simulink model "Aircraft6dof_V2"  (R2025b)
settings: Solver=ode4  StartTime=startTime  StopTime=A8.stopTime  FixedStep=stepTime  RelTol=1e-3  EnableMultiTasking=on
undefined symbols (not defined in the file): a0_s2, a0_s3, a0_s4, a0_s5, A8, AR_s2, AR_s3, AR_s4, AR_s5, ARvecP1, Att_Trim, c_s2, c_s3, c_s4, c_s5, CD0_s2, CD0_s3, CD0_s4, CD0_s5, CDa_s2, CDa_s3, CDa_s4, CDa_s5, CL0_s2, CL0_s3, CL0_s4, CL0_s5, CM0_s2, CM0_s3, CM0_s4, CM0_s5, CMa_s2, CMa_s3, CMa_s4, CMa_s5, CQvecP1, CTvecP1, dCL_du, e_s2, e_s3, e_s4, e_s5, i_s2, i_s3, i_s4, i_s5, InitAtt, J, J_int, K_lqr_cmd, m, n_int, n_p1, n_s2, n_s3, n_s4, n_s5, R_p1, Rates_Trim, S_s2 ... (+15)
libraries: vrlib x9, simulink x5
(part 1 of 3)
settings Model: Creator=McArthur  LastModifiedBy=jacks
settings SolverCC: AlgebraicLoopSolver=TrustRegion
settings DataIOCC: LimitDataPoints=on  SaveFormat=StructureWithTime  ReturnWorkspaceOutputs=off
settings OptimizationCC: LifeSpan=inf
settings DebuggingCC: UnconnectedInputMsg=warning  UnconnectedOutputMsg=warning  UnconnectedLineMsg=warning  SFUnexpectedBacktrackingDiag=warning  SFNoUnconditionalDefaultTransitionDiag=warning  SFExecutionAtInitializationDiag=none  ArithmeticOperatorsInVariantConditions=warning
settings HardwareCC: ProdBitPerSizeT=32.0  ProdBitPerPtrDiffT=32.0  ProdWordSize=32.0  ProdHWDeviceType=Specified
settings ModelReferenceCC: EnableRefExpFcnMdlSchedulingChecks=on  PropagateSignalLabelsOutOfModel=off
settings SFSimCC: SimUseLocalCustomCode=off  CustomCodeUndefinedFunction=UseInterfaceOnly
settings RTWCC: RTWUseLocalCustomCode=off  GPUComputeCapability=3.5
settings CodeAppCC: StateflowObjectComments=on
settings GRTTargetCC: TargetLangStandard=C89/C90 (ANSI)
settings ConfigComp: CovMetricSettings=dw  CovSaveCumulativeToWorkspaceVar=on  CovSaveSingleToWorkspaceVar=on  CovExternalEMLEnable=off

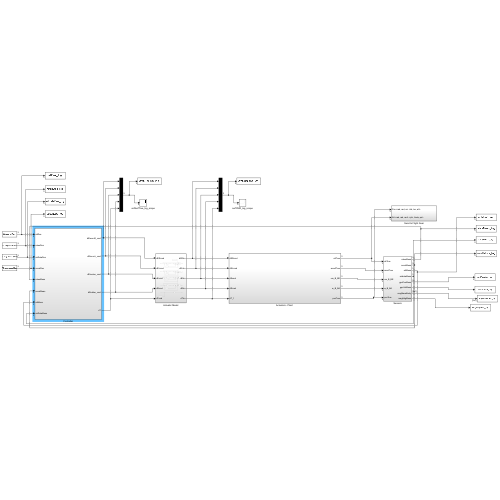
[thumbnail: Simulink's stored preview of the top-level diagram]
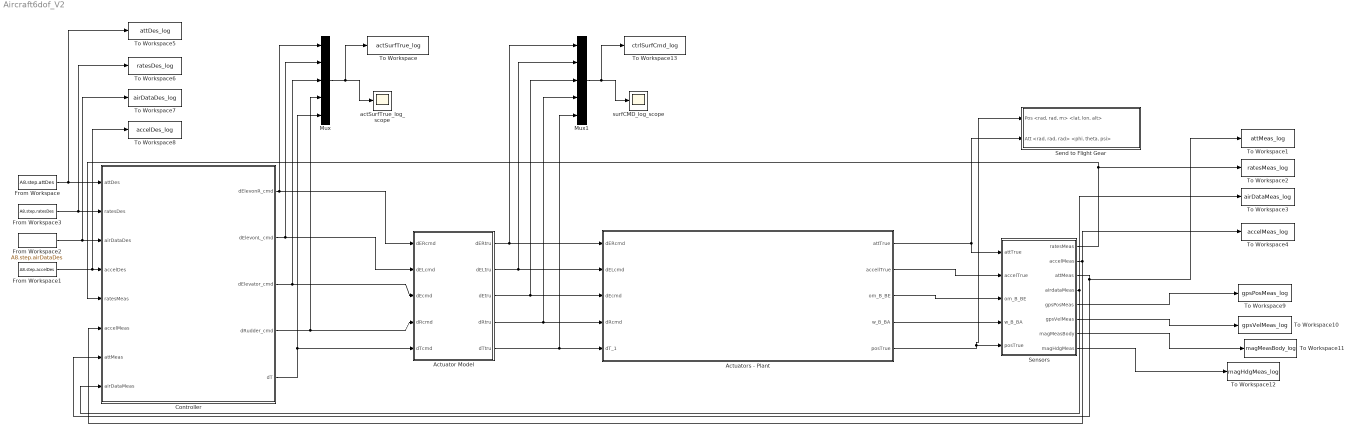
== system Aircraft6dof_V2 ==
  Actuator Model : Subsystem
  "Actuators - Plant " : Subsystem
  Controller : Subsystem
  From Workspace : FromWorkspace  VariableName=A8.step.attDes
  From Workspace1 : FromWorkspace  VariableName=A8.step.accelDes
  From Workspace2 : FromWorkspace  VariableName=A8.step.airDataDes
  From Workspace3 : FromWorkspace  VariableName=A8.step.ratesDes
  Mux : Mux  Inputs=5
  Mux1 : Mux  Inputs=5
  Send to Flight Gear : Subsystem
  Sensors : Subsystem
  To Workspace : ToWorkspace  VariableName=actSurfTrue_log  SaveFormat=Timeseries  SampleTime=-1
  To Workspace1 : ToWorkspace  VariableName=attMeas_log  SaveFormat=Timeseries  SampleTime=-1
  To Workspace10 : ToWorkspace  VariableName=gpsVelMeas_log  SaveFormat=Timeseries  SampleTime=-1
  To Workspace11 : ToWorkspace  VariableName=magMeasBody_log  SaveFormat=Timeseries  SampleTime=-1
  To Workspace12 : ToWorkspace  VariableName=magHdgMeas_log  SaveFormat=Timeseries  SampleTime=-1
  To Workspace13 : ToWorkspace  VariableName=ctrlSurfCmd_log  SaveFormat=Timeseries  SampleTime=-1
  To Workspace2 : ToWorkspace  VariableName=ratesMeas_log  SaveFormat=Timeseries  SampleTime=-1
  To Workspace3 : ToWorkspace  VariableName=airDataMeas_log  SaveFormat=Timeseries  SampleTime=-1
  To Workspace4 : ToWorkspace  VariableName=accelMeas_log  SaveFormat=Timeseries  SampleTime=-1
  To Workspace5 : ToWorkspace  VariableName=attDes_log  SaveFormat=Timeseries  SampleTime=-1
  To Workspace6 : ToWorkspace  VariableName=ratesDes_log  SaveFormat=Timeseries  SampleTime=-1
  To Workspace7 : ToWorkspace  VariableName=airDataDes_log  SaveFormat=Timeseries  SampleTime=-1
  To Workspace8 : ToWorkspace  VariableName=accelDes_log  SaveFormat=Timeseries  SampleTime=-1
  To Workspace9 : ToWorkspace  VariableName=gpsPosMeas_log  SaveFormat=Timeseries  SampleTime=-1
  actSurfTrue_log_scope : Scope
      settings: ActiveDisplayYMinimum=-0.54541539124822791  ActiveDisplayYMaximum=0.54541539124822791  DataLoggingVariableName=ScopeData24
  surfCMD_log_scope : Scope
      settings: ActiveDisplayYMinimum=-0.54541539124822791  ActiveDisplayYMaximum=0.54541539124822791  DataLoggingVariableName=ScopeData12
  wires:
  "Actuators - Plant "/5(posTrue) -> Send to Flight Gear/1("Pos <rad, rad, m> <lat, lon, alt>"), Sensors/5(posTrue)
  "Actuators - Plant "/4(w_B_BA) -> Sensors/4(w_B_BA)
  "Actuators - Plant "/3(om_B_BE) -> Sensors/3(om_B_BE)
  "Actuators - Plant "/2(accellTrue) -> Sensors/2(accelTrue)
  "Actuators - Plant "/1(attTrue) -> Send to Flight Gear/2("Att <rad, rad, rad> <phi, theta, psi>"), Sensors/1(attTrue)
  Controller/4(dRudder_cmd) -> Actuator Model/4(dRcmd), Mux/4
  Controller/3(dElevator_cmd) -> Actuator Model/3(dEcmd), Mux/3
  Controller/2(dElevonL_cmd) -> Actuator Model/2(dELcmd), Mux/2
  Controller/1(dElevonR_cmd) -> Actuator Model/1(dERcmd), Mux/1
  Sensors/1(ratesMeas) -> To Workspace2/1, Controller/5(ratesMeas)
  Sensors/3(attMeas) -> To Workspace1/1, Controller/7(attMeas)
  Sensors/2(accelMeas) -> Controller/6(accelMeas), To Workspace4/1
  Sensors/4(airdataMeas) -> Controller/8(airDataMeas), To Workspace3/1
  From Workspace1/1 -> To Workspace8/1, Controller/4(accelDes)
  From Workspace2/1 -> To Workspace7/1, Controller/3(airDataDes)
  From Workspace3/1 -> To Workspace6/1, Controller/2(ratesDes)
  Mux/1 -> actSurfTrue_log_scope/1, To Workspace/1
  Sensors/5(gpsPosMeas) -> To Workspace9/1
  Sensors/6(gpsVelMeas) -> To Workspace10/1
  Sensors/7(magMeasBody) -> To Workspace11/1
  Sensors/8(magHdgMeas) -> To Workspace12/1
  From Workspace/1 -> To Workspace5/1, Controller/1(attDes)
  Actuator Model/1(dERtru) -> Mux1/1, "Actuators - Plant "/1(dERcmd)
  Actuator Model/2(dELtru) -> Mux1/2, "Actuators - Plant "/2(dELcmd)
  Actuator Model/3(dEtru) -> Mux1/3, "Actuators - Plant "/3(dEcmd)
  Actuator Model/4(dRtru) -> Mux1/4, "Actuators - Plant "/4(dRcmd)
  Actuator Model/5(dTtru) -> Mux1/5, "Actuators - Plant "/5(dT_1)
  Controller/5(dT) -> Mux/5, Actuator Model/5(dTcmd)
  Mux1/1 -> surfCMD_log_scope/1, To Workspace13/1

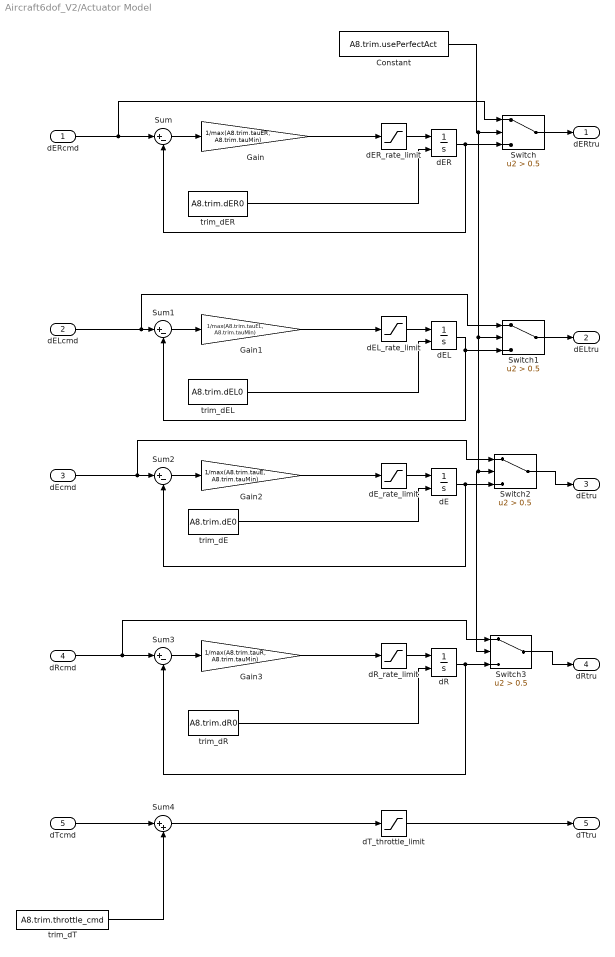
== system Aircraft6dof_V2/Actuator Model ==
  dERcmd : Inport
  dELcmd : Inport  Port=2
  dEcmd : Inport  Port=3
  dRcmd : Inport  Port=4
  dTcmd : Inport  Port=5
  Constant : Constant  Value=A8.trim.usePerfectAct
  Gain : Gain  Gain=1/max(A8.trim.tauER, A8.trim.tauMin)
  Gain1 : Gain  Gain=1/max(A8.trim.tauEL, A8.trim.tauMin)
  Gain2 : Gain  Gain=1/max(A8.trim.tauE, A8.trim.tauMin)
  Gain3 : Gain  Gain=1/max(A8.trim.tauR, A8.trim.tauMin)
  Sum{,1..3} (4 alike) : Sum  Inputs=|+-
  Sum4 : Sum  Inputs=|++
  Switch{,1..3} (4 alike) : Switch  Criteria=u2 > Threshold  Threshold=0.5  SaturateOnIntegerOverflow=off  InputSameDT=off
  dE : Integrator  InitialConditionSource=external  LimitOutput=on  UpperSaturationLimit=A8.trim.dE_max  LowerSaturationLimit=A8.trim.dE_min
  dEL : Integrator  InitialConditionSource=external  LimitOutput=on  UpperSaturationLimit=A8.trim.dEL_max  LowerSaturationLimit=A8.trim.dEL_min
  dEL_rate_limit : Saturate  UpperLimit=A8.trim.dELdot_max  LowerLimit=-A8.trim.dELdot_max
  dER : Integrator  InitialConditionSource=external  LimitOutput=on  UpperSaturationLimit=A8.trim.dER_max  LowerSaturationLimit=A8.trim.dER_min
  dER_rate_limit : Saturate  UpperLimit=A8.trim.dERdot_max  LowerLimit=-A8.trim.dERdot_max
  dE_rate_limit : Saturate  UpperLimit=A8.trim.dEdot_max  LowerLimit=-A8.trim.dEdot_max
  dR : Integrator  InitialConditionSource=external  LimitOutput=on  UpperSaturationLimit=A8.trim.dR_max  LowerSaturationLimit=A8.trim.dR_min
  dR_rate_limit : Saturate  UpperLimit=A8.trim.dRdot_max  LowerLimit=-A8.trim.dRdot_max
  dT_throttle_limit : Saturate  UpperLimit=A8.trim.dT1_max  LowerLimit=A8.trim.dT1_min
  trim_dE : Constant  Value=A8.trim.dE0
  trim_dEL : Constant  Value=A8.trim.dEL0
  trim_dER : Constant  Value=A8.trim.dER0
  trim_dR : Constant  Value=A8.trim.dR0
  trim_dT : Constant  Value=A8.trim.throttle_cmd
  dERtru : Outport  VectorParamsAs1DForOutWhenUnconnected=off
  dELtru : Outport  Port=2  VectorParamsAs1DForOutWhenUnconnected=off
  dEtru : Outport  Port=3  VectorParamsAs1DForOutWhenUnconnected=off
  dRtru : Outport  Port=4  VectorParamsAs1DForOutWhenUnconnected=off
  dTtru : Outport  Port=5
  wires:
  trim_dR/1 -> dR/2
  dER/1 -> Switch/3, Sum/2
  dE/1 -> Switch2/3, Sum2/2
  trim_dER/1 -> dER/2
  Gain1/1 -> dEL_rate_limit/1
  dERcmd/1 -> Switch/1, Sum/1
  Sum2/1 -> Gain2/1
  trim_dEL/1 -> dEL/2
  Gain/1 -> dER_rate_limit/1
  Gain3/1 -> dR_rate_limit/1
  trim_dE/1 -> dE/2
  dRcmd/1 -> Switch3/1, Sum3/1
  Gain2/1 -> dE_rate_limit/1
  Sum1/1 -> Gain1/1
  Sum/1 -> Gain/1
  Sum3/1 -> Gain3/1
  dELcmd/1 -> Switch1/1, Sum1/1
  dEcmd/1 -> Switch2/1, Sum2/1
  dEL/1 -> Switch1/3, Sum1/2
  dR/1 -> Switch3/3, Sum3/2
  dT_throttle_limit/1 -> dTtru/1
  dTcmd/1 -> Sum4/1
  trim_dT/1 -> Sum4/2
  dER_rate_limit/1 -> dER/1
  dEL_rate_limit/1 -> dEL/1
  dE_rate_limit/1 -> dE/1
  dR_rate_limit/1 -> dR/1
  Sum4/1 -> dT_throttle_limit/1
  Switch/1 -> dERtru/1
  Constant/1 -> Switch3/2, Switch2/2, Switch1/2, Switch/2
  Switch1/1 -> dELtru/1
  Switch2/1 -> dEtru/1
  Switch3/1 -> dRtru/1

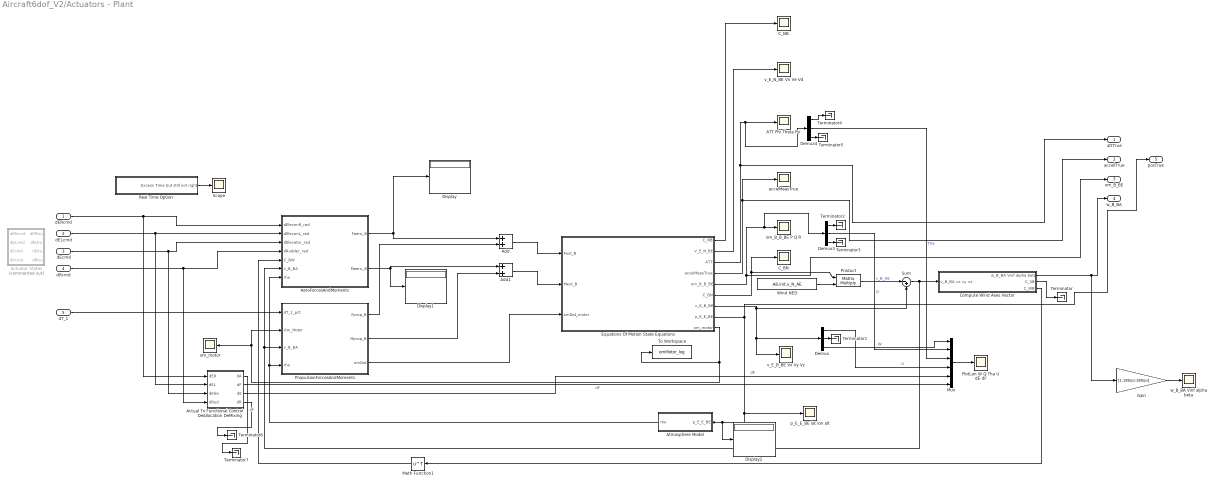
== system Aircraft6dof_V2/Actuators - Plant  ==
  dERcmd : Inport
  dELcmd : Inport  Port=2
  dEcmd : Inport  Port=3
  dRcmd : Inport  Port=4
  dT_1 : Inport  Port=5
  ATT Phi Theta Psi : Scope
      settings: TimeSpan=100  ActiveDisplayYMinimum=-0.03536052016506628  ActiveDisplayYMaximum=0.060071284999749723  DataLoggingVariableName=ScopeData6
  Actual To Functional Control DeAllocation DeMixing : Subsystem
  Actuator States : Subsystem  Commented=on
  Add : Sum
  Add1 : Sum
  AeroForcesAndMoments : Subsystem
  Atmosphere Model : Subsystem
  C_BN : Scope
      settings: ActiveDisplayYMinimum=-1.25  ActiveDisplayYMaximum=1.25  DataLoggingVariableName=ScopeData7
  C_NB : Scope
      settings: DataLoggingVariableName=ScopeData8  DataLoggingSaveFormat=Array
  Compute Wind Axes Vector : Subsystem
  Demux : Demux  Outputs=3
  Demux3 : Demux  Outputs=3
  Demux4 : Demux  Outputs=3
  Display : Display
  Display1 : Display
  Display2 : Display
  Equations Of Motion State Equations : Subsystem
  Gain : Gain  Gain=[1;180/pi;180/pi]
  Math Function1 : Math  Operator=transpose  SignedPower=on
  Mux : Mux  Inputs=6
  PlotLon W Q Tha U dE dF : Scope
      settings: TimeSpan=100  ActiveDisplayYMinimum=-109.39087703202826  ActiveDisplayYMaximum=114.84829731514765  DataLoggingVariableName=ScopeData11
  Product : Product  Multiplication=Matrix(*)
  PropulsionForcesAndMoments : Subsystem
  Real Time Option : Subsystem
  Scope : Scope
      settings: ActiveDisplayYMinimum=-0.02501  ActiveDisplayYMaximum=0.00268
  Sum : Sum  Inputs=|-+
  Terminator{,1..7} (8 alike) : Terminator
  To Workspace : ToWorkspace  VariableName=omMotor_log  SaveFormat=Timeseries  SampleTime=-1
  Wind NED : Constant  Value=A8.init.v_N_AE
  accelMeasTrue : Scope
      settings: TimeSpan=20  ActiveDisplayYMinimum=-12  ActiveDisplayYMaximum=3  DataLoggingVariableName=ScopeData5  DataLoggingSaveFormat=Array
  om_B_B_BE P Q R : Scope
      settings: TimeSpan=20  ActiveDisplayYMinimum=-0.175  ActiveDisplayYMaximum=0.125  DataLoggingVariableName=ScopeData4
  om_motor : Scope
      settings: TimeSpan=20  ActiveDisplayYMinimum=-1  ActiveDisplayYMaximum=1  DataLoggingVariableName=ScopeData2
  p_E_E_BE lat lon alt : Scope
      settings: ActiveDisplayYMinimum=-2197.24995  ActiveDisplayYMaximum=255.24999
  v_E_B_BE Vx Vy Vz : Scope
      settings: TimeSpan=20  ActiveDisplayYMinimum=-95.74229  ActiveDisplayYMaximum=24.82944  DataLoggingVariableName=ScopeData3
  v_E_N_BE Vn Ve Vd : Scope
      settings: TimeSpan=20  ActiveDisplayYMinimum=-27.392800404423681  ActiveDisplayYMaximum=39.4717463834183  DataLoggingVariableName=ScopeData9  DataLoggingSaveFormat=Array
  w_B_BA Vinf alpha beta : Scope
      settings: TimeSpan=20  ActiveDisplayYMinimum=-1  ActiveDisplayYMaximum=1  DataLoggingVariableName=ScopeData10
  attTrue : Outport
  accellTrue : Outport  Port=2
  om_B_BE : Outport  Port=3
  w_B_BA : Outport  Port=4
  posTrue : Outport  Port=5
  wires:
  Real Time Option/1(Excess Time but still not right) -> Scope/1
  AeroForcesAndMoments/2(Maero_B) -> Add1/1, Display1/1
  PropulsionForcesAndMoments/3(omDot) -> Equations Of Motion State Equations/3(omDot_motor)
  AeroForcesAndMoments/1(Faero_B) -> Add/1, Display/1
  Equations Of Motion State Equations/8(p_E_E_BE) -> Display2/1, Atmosphere Model/1(p_E_E_BE), p_E_E_BE lat lon alt/1, posTrue/1
  Equations Of Motion State Equations/2(V_E_N_BE) -> v_E_N_BE Vn Ve Vd/1
  Equations Of Motion State Equations/1(C_NB) -> C_NB/1
  Sum/1 -> PropulsionForcesAndMoments/3(v_B_BA), AeroForcesAndMoments/6(v_B_BA), Compute Wind Axes Vector/1(v_B_BA vx vy vz)
  Compute Wind Axes Vector/3(C_WB) -> Math Function1/1
  Math Function1/1 -> AeroForcesAndMoments/5(C_BW)
  Equations Of Motion State Equations/5(om_B_B_BE) -> Demux3/1, om_B_B_BE P Q R/1, om_B_BE/1
  Equations Of Motion State Equations/6(C_BN) -> C_BN/1, Product/1
  Product/1 -> Sum/1  "v_B_AE"
  Gain/1 -> w_B_BA Vinf alpha beta/1
  Atmosphere Model/1(rho) -> PropulsionForcesAndMoments/4(rho), AeroForcesAndMoments/7(rho)
  Compute Wind Axes Vector/1(w_B_BA Vinf alpha beta) -> Gain/1, w_B_BA/1
  Compute Wind Axes Vector/2(C_SB) -> Terminator/1
  Equations Of Motion State Equations/7(v_E_B_BE) -> Sum/2, v_E_B_BE Vx Vy Vz/1, Demux/1
  Equations Of Motion State Equations/4(accelMeasTrue) -> accellTrue/1, accelMeasTrue/1
  Wind NED/1 -> Product/2
  Mux/1 -> PlotLon W Q Tha U dE dF/1
  Demux/3 -> Mux/1  "W"
  Demux/1 -> Mux/4  "U"
  Demux/2 -> Terminator1/1
  Demux3/2 -> Mux/2  "Q"
  Demux3/1 -> Terminator2/1
  Demux3/3 -> Terminator3/1
  Equations Of Motion State Equations/3(ATT) -> Demux4/1, ATT Phi Theta Psi/1, attTrue/1
  Demux4/2 -> Mux/3  "Tha"
  Demux4/1 -> Terminator4/1
  Demux4/3 -> Terminator5/1
  Actual To Functional Control DeAllocation DeMixing/3(dE) -> Mux/5  "dE"
  Actual To Functional Control DeAllocation DeMixing/2(dF) -> Mux/6  "dF"
  Add/1 -> Equations Of Motion State Equations/1(Fext_B)
  Add1/1 -> Equations Of Motion State Equations/2(Mext_B)
  dT_1/1 -> PropulsionForcesAndMoments/1(dT_1_pct)
  PropulsionForcesAndMoments/1(Fprop_B) -> Add/2
  PropulsionForcesAndMoments/2(Mprop_B) -> Add1/2
  Equations Of Motion State Equations/9(om_motor) -> To Workspace/1, PropulsionForcesAndMoments/2(Om_Motor), om_motor/1
  Actual To Functional Control DeAllocation DeMixing/4(dR) -> Terminator6/1
  Actual To Functional Control DeAllocation DeMixing/1(dA) -> Terminator7/1  "dF"
  dERcmd/1 -> Actual To Functional Control DeAllocation DeMixing/1(dER), AeroForcesAndMoments/1(dElevonR_rad)
  dELcmd/1 -> Actual To Functional Control DeAllocation DeMixing/2(dEL), AeroForcesAndMoments/2(dElevonL_rad)
  dEcmd/1 -> Actual To Functional Control DeAllocation DeMixing/3(dElev), AeroForcesAndMoments/3(dElevator_rad)
  dRcmd/1 -> Actual To Functional Control DeAllocation DeMixing/4(dRud), AeroForcesAndMoments/4(dRudder_rad)

== system Aircraft6dof_V2/Controller ==
  attDes : Inport
  ratesDes : Inport  Port=2
  airDataDes : Inport  Port=3
  accelDes : Inport  Port=4
  ratesMeas : Inport  Port=5
  accelMeas : Inport  Port=6
  attMeas : Inport  Port=7
  airDataMeas : Inport  Port=8
  Constant1 : Constant  Value=A8.gains.on
  ControlMixer_A8 : Subsystem
  Demux : Demux  Outputs=5
  LQR Controller : Subsystem
  Multiport Switch : MultiPortSwitch  SaturateOnIntegerOverflow=off  InputSameDT=off
  Mux : Mux  Inputs=5
  Mux1 : Mux  Inputs=5
  Mux2 : Mux  Inputs=5
  "No Feedback Open Loop Commands Steps, Ramps, Sweeps, etc" : Subsystem
  PID Controller : Subsystem
  To Workspace : ToWorkspace  VariableName=ctrlFunc_log  SaveFormat=Timeseries  SampleTime=-1
  dElevonR_cmd : Outport  VectorParamsAs1DForOutWhenUnconnected=off
  dElevonL_cmd : Outport  Port=2  VectorParamsAs1DForOutWhenUnconnected=off
  dElevator_cmd : Outport  Port=3  VectorParamsAs1DForOutWhenUnconnected=off
  dRudder_cmd : Outport  Port=4  VectorParamsAs1DForOutWhenUnconnected=off
  dT : Outport  Port=5  VectorParamsAs1DForOutWhenUnconnected=off
  wires:
  accelMeas/1 -> "No Feedback Open Loop Commands Steps, Ramps, Sweeps, etc"/8(accelMeas), PID Controller/8(accelMeas)
  attDes/1 -> LQR Controller/4(attDes), PID Controller/1(attDes), "No Feedback Open Loop Commands Steps, Ramps, Sweeps, etc"/1(attDes)
  ratesMeas/1 -> LQR Controller/2(ratesMeas), "No Feedback Open Loop Commands Steps, Ramps, Sweeps, etc"/6(ratesMeas), PID Controller/6(ratesMeas)
  ratesDes/1 -> LQR Controller/5(ratesDes), "No Feedback Open Loop Commands Steps, Ramps, Sweeps, etc"/2(ratesDes), PID Controller/2(ratesDes)
  attMeas/1 -> LQR Controller/1(attMeas), "No Feedback Open Loop Commands Steps, Ramps, Sweeps, etc"/5(attMeas), PID Controller/5(attMeas)
  Demux/1 -> ControlMixer_A8/1(dA)
  airDataDes/1 -> LQR Controller/6(airDataDes), "No Feedback Open Loop Commands Steps, Ramps, Sweeps, etc"/3(airDataDes), PID Controller/3(airDataDes)
  accelDes/1 -> "No Feedback Open Loop Commands Steps, Ramps, Sweeps, etc"/4(accelDes), PID Controller/4(accelDes)
  airDataMeas/1 -> LQR Controller/3(airDataMeas), "No Feedback Open Loop Commands Steps, Ramps, Sweeps, etc"/7(airDataMeas), PID Controller/7(airDataMeas)
  ControlMixer_A8/2(dELcmd) -> dElevonL_cmd/1
  "No Feedback Open Loop Commands Steps, Ramps, Sweeps, etc"/1(dAil) -> Mux/1
  "No Feedback Open Loop Commands Steps, Ramps, Sweeps, etc"/4(dRud) -> Mux/4
  "No Feedback Open Loop Commands Steps, Ramps, Sweeps, etc"/3(dElev) -> Mux/3
  "No Feedback Open Loop Commands Steps, Ramps, Sweeps, etc"/2(dFlap) -> Mux/2
  "No Feedback Open Loop Commands Steps, Ramps, Sweeps, etc"/5(dT) -> Mux/5
  PID Controller/4(dRud) -> Mux1/4
  PID Controller/3(dElev) -> Mux1/3
  PID Controller/2(dFlap) -> Mux1/2
  PID Controller/1(dAil) -> Mux1/1
  PID Controller/5(dT) -> Mux1/5
  Mux/1 -> Multiport Switch/2
  Demux/5 -> ControlMixer_A8/5(dT)
  Demux/4 -> ControlMixer_A8/4(dR)
  Demux/3 -> ControlMixer_A8/3(dE)
  Demux/2 -> ControlMixer_A8/2(dF)
  ControlMixer_A8/1(dERcmd) -> dElevonR_cmd/1
  ControlMixer_A8/3(dElevcmd) -> dElevator_cmd/1
  ControlMixer_A8/4(dRudcmd) -> dRudder_cmd/1
  ControlMixer_A8/5(dTcmd) -> dT/1
  Constant1/1 -> Multiport Switch/1
  Mux1/1 -> Multiport Switch/3
  LQR Controller/4(dRud) -> Mux2/4
  LQR Controller/5(dT) -> Mux2/5
  LQR Controller/3(dElev) -> Mux2/3
  LQR Controller/2(dFlap) -> Mux2/2
  LQR Controller/1(dAil) -> Mux2/1
  Mux2/1 -> Multiport Switch/4
  Multiport Switch/1 -> To Workspace/1, Demux/1

== system Aircraft6dof_V2/Send to Flight Gear ==
  "Pos <rad, rad, m> <lat, lon, alt>" : Inport
  "Att <rad, rad, rad> <phi, theta, psi>" : Inport  Port=2
  S-Function : S-Function  FunctionName=sfun_FlightGearSender  Parameters=stepTime, '127.0.0.1', 5502  SFunctionDeploymentMode=off  EnableBusSupport=off
  wires:
  "Pos <rad, rad, m> <lat, lon, alt>"/1 -> S-Function/1
  "Att <rad, rad, rad> <phi, theta, psi>"/1 -> S-Function/2

== system Aircraft6dof_V2/Sensors ==
  attTrue : Inport
  accelTrue : Inport  Port=2
  om_B_BE : Inport  Port=3
  w_B_BA : Inport  Port=4
  posTrue : Inport  Port=5
  AccelSensor : Subsystem
  AirDataSensor : Subsystem
  AttitudeSensor : Subsystem
  GPSSensor : Subsystem
  GyroSensor : Subsystem
  MagSensor : Subsystem
  Selector : Selector  InputPortWidth=3  IndexOptions=Index vector (dialog)  Indices=[1]  OutputSizes=1
  ratesMeas : Outport  VectorParamsAs1DForOutWhenUnconnected=off
  accelMeas : Outport  Port=2  VectorParamsAs1DForOutWhenUnconnected=off
  attMeas : Outport  Port=3  VectorParamsAs1DForOutWhenUnconnected=off
  airdataMeas : Outport  Port=4
  gpsPosMeas : Outport  Port=5
  gpsVelMeas : Outport  Port=6
  magMeasBody : Outport  Port=7
  magHdgMeas : Outport  Port=8
  wires:
  AccelSensor/1(accelMeas) -> accelMeas/1
  accelTrue/1 -> AccelSensor/1(accelTrue)
  attTrue/1 -> AttitudeSensor/1(attTrue), MagSensor/1(attTrue)
  GyroSensor/1(ratesMeas) -> ratesMeas/1
  Selector/1 -> GPSSensor/2(velTrue)
  w_B_BA/1 -> AirDataSensor/1(w_B_BA), Selector/1
  om_B_BE/1 -> GyroSensor/1(ratesTrue)
  AttitudeSensor/1(attMeas) -> attMeas/1
  MagSensor/1(magMeasBody) -> magMeasBody/1
  MagSensor/2(magHdgMeas) -> magHdgMeas/1
  posTrue/1 -> GPSSensor/1(posTrue)
  AirDataSensor/1(airdataMeas) -> airdataMeas/1
  GPSSensor/2(gpsVelMeas) -> gpsVelMeas/1
  GPSSensor/1(gpsPosMeas) -> gpsPosMeas/1

== system Aircraft6dof_V2/Actuators - Plant /Actual To Functional Control DeAllocation DeMixing ==
  dER : Inport
  dEL : Inport  Port=2
  dElev : Inport  Port=3
  dRud : Inport  Port=4
  Constant1 : Constant  Value=A8.trim.DeMixMatrix
  Demux : Demux
  Mux : Mux
  Product1 : Product  Multiplication=Matrix(*)
  dA : Outport  VectorParamsAs1DForOutWhenUnconnected=off
  dF : Outport  Port=2  VectorParamsAs1DForOutWhenUnconnected=off
  dE : Outport  Port=3  VectorParamsAs1DForOutWhenUnconnected=off
  dR : Outport  Port=4  VectorParamsAs1DForOutWhenUnconnected=off
  wires:
  dER/1 -> Mux/1
  dEL/1 -> Mux/2
  dElev/1 -> Mux/3
  dRud/1 -> Mux/4
  Demux/2 -> dF/1
  Constant1/1 -> Product1/1
  Mux/1 -> Product1/2
  Demux/1 -> dA/1
  Demux/4 -> dR/1
  Demux/3 -> dE/1
  Product1/1 -> Demux/1

== system Aircraft6dof_V2/Actuators - Plant /Actuator States ==
  dERcmd : Inport
  dELcmd : Inport  Port=2
  dEcmd : Inport  Port=3
  dRcmd : Inport  Port=4
  Gain : Gain  Gain=1/A8.trim.tauER
  Gain1 : Gain  Gain=1/A8.trim.tauEL
  Gain2 : Gain  Gain=1/A8.trim.tauE
  Gain3 : Gain  Gain=1/A8.trim.tauR
  Sum{,1..3} (4 alike) : Sum  Inputs=|+-
  dE : Integrator  InitialConditionSource=external
  dEL : Integrator  InitialConditionSource=external
  dER : Integrator  InitialConditionSource=external
  dR : Integrator  InitialConditionSource=external
  trim_dE : Constant  Value=A8.trim.dE0
  trim_dEL : Constant  Value=A8.trim.dEL0
  trim_dER : Constant  Value=A8.trim.dER0
  trim_dR : Constant  Value=A8.trim.dR0
  dERtru : Outport  VectorParamsAs1DForOutWhenUnconnected=off
  dELtru : Outport  Port=2  VectorParamsAs1DForOutWhenUnconnected=off
  dEtru : Outport  Port=3  VectorParamsAs1DForOutWhenUnconnected=off
  dRtru : Outport  Port=4  VectorParamsAs1DForOutWhenUnconnected=off
  wires:
  dER/1 -> Sum/2, dERtru/1
  dERcmd/1 -> Sum/1
  Gain/1 -> dER/1
  Sum/1 -> Gain/1
  trim_dER/1 -> dER/2
  dEL/1 -> Sum1/2, dELtru/1
  dELcmd/1 -> Sum1/1
  Gain1/1 -> dEL/1
  Sum1/1 -> Gain1/1
  trim_dEL/1 -> dEL/2
  dE/1 -> Sum2/2, dEtru/1
  dEcmd/1 -> Sum2/1
  Gain2/1 -> dE/1
  Sum2/1 -> Gain2/1
  trim_dE/1 -> dE/2
  dR/1 -> Sum3/2, dRtru/1
  dRcmd/1 -> Sum3/1
  Gain3/1 -> dR/1
  Sum3/1 -> Gain3/1
  trim_dR/1 -> dR/2

== system Aircraft6dof_V2/Actuators - Plant /AeroForcesAndMoments ==
  dElevonR_rad : Inport
  dElevonL_rad : Inport  Port=2
  dElevator_rad : Inport  Port=3
  dRudder_rad : Inport  Port=4
  C_BW : Inport  Port=5
  v_B_BA : Inport  Port=6
  rho : Inport  Port=7
  Add : Sum  Inputs=++++
  Add1 : Sum  Inputs=++++
  Display1 : Display
  Display3 : Display
  Surface2 : Subsystem
  Surface3 : Subsystem
  Surface4 : Subsystem
  Surface5 : Subsystem
  Faero_B : Outport  VectorParamsAs1DForOutWhenUnconnected=off
  Maero_B : Outport  Port=2  VectorParamsAs1DForOutWhenUnconnected=off
  wires:
  C_BW/1 -> Surface2/1(C_BW), Surface3/1(C_BW), Surface5/1(C_BW), Surface4/1(C_BW)
  v_B_BA/1 -> Surface3/2(v_B_BA), Surface2/2(v_B_BA), Surface5/2(v_B_BA), Surface4/2(v_B_BA)
  rho/1 -> Surface3/3(rho), Surface2/3(rho), Surface5/3(rho), Surface4/3(rho)
  Surface4/1(Fs4_B) -> Add/1
  Surface5/1(Fs5_B) -> Add/2
  Surface4/2(Ms4_B) -> Add1/1
  Surface5/2(Ms5_B) -> Add1/2
  Surface2/1(Fs2_B) -> Add/3
  Surface2/2(Ms2_B) -> Add1/3
  Add1/1 -> Display1/1, Maero_B/1
  Add/1 -> Display3/1, Faero_B/1
  Surface3/1(Fs2_B) -> Add/4
  Surface3/2(Ms2_B) -> Add1/4
  dElevonR_rad/1 -> Surface4/4(u_s#_rad)
  dElevonL_rad/1 -> Surface5/4(u_s#_rad)
  dElevator_rad/1 -> Surface2/4(u_s#_rad)
  dRudder_rad/1 -> Surface3/4(u_s#_rad)

== system Aircraft6dof_V2/Actuators - Plant /Atmosphere Model ==
  p_E_E_BE : Inport
  Compare To Constant : simulink/Logic and Bit Operations/Compare To Constant  relop=<=  const=11000  OutDataTypeStr=boolean
  Demux : Demux  Outputs=3
  Enhance Me Please! : Constant  Value=0
  Standard Atmosphere - Troposphere : MATLAB Function  TreatAsAtomicUnit=on
  Switch : Switch  Criteria=u2 ~= 0  Threshold=11000  SaturateOnIntegerOverflow=off  InputSameDT=off
  Terminator : Terminator
  Terminator1 : Terminator
  rho : Outport  VectorParamsAs1DForOutWhenUnconnected=off
  wires:
  p_E_E_BE/1 -> Demux/1
  Demux/1 -> Terminator/1
  Demux/2 -> Terminator1/1
  Demux/3 -> Standard Atmosphere - Troposphere/1(h), Compare To Constant/1
  Compare To Constant/1 -> Switch/2
  Standard Atmosphere - Troposphere/1(rho) -> Switch/1
  Switch/1 -> rho/1
  Enhance Me Please!/1 -> Switch/3

== system Aircraft6dof_V2/Actuators - Plant /Compute Wind Axes Vector ==
  v_B_BA vx vy vz : Inport
  Compute Wind DCMs : MATLAB Function  TreatAsAtomicUnit=on
  Constant : Constant  Value=[0;0;0]
  Constant1 : Constant  Value=0.001
  Demux : Demux  Outputs=3
  Display : Display
  Divide : Product  Inputs=*/
  Dot Product : DotProduct  OutDataTypeStr=Inherit: Inherit via internal rule
  MinMax : MinMax  Function=max  Inputs=2
  Mux : Mux  Inputs=3
  Saturation : Saturate  UpperLimit=1  LowerLimit=-1
  Sqrt : Sqrt
  Switch : Switch  Criteria=u2 > Threshold  SaturateOnIntegerOverflow=off  InputSameDT=off
  Trigonometric Function : Trigonometry  Operator=atan2
  Trigonometric Function1 : Trigonometry  Operator=asin
  w_B_BA Vinf alpha beta : Outport  VectorParamsAs1DForOutWhenUnconnected=off
  C_SB : Outport  Port=2  VectorParamsAs1DForOutWhenUnconnected=off
  C_WB : Outport  Port=3  VectorParamsAs1DForOutWhenUnconnected=off
  wires:
  Dot Product/1 -> Sqrt/1
  Mux/1 -> Switch/1
  Constant/1 -> Switch/3
  Trigonometric Function/1 -> Display/1, Compute Wind DCMs/2(alpha), Mux/2
  Switch/1 -> w_B_BA Vinf alpha beta/1
  Demux/3 -> Trigonometric Function/1
  v_B_BA vx vy vz/1 -> Demux/1, Dot Product/2, Dot Product/1
  Demux/1 -> Trigonometric Function/2
  Constant1/1 -> MinMax/1
  MinMax/1 -> Divide/2
  Demux/2 -> Divide/1
  Divide/1 -> Saturation/1
  Saturation/1 -> Trigonometric Function1/1
  Trigonometric Function1/1 -> Compute Wind DCMs/3(beta), Mux/3
  Sqrt/1 -> Compute Wind DCMs/1(Vinf), Mux/1, Switch/2, MinMax/2
  Compute Wind DCMs/2(C_WB) -> C_WB/1
  Compute Wind DCMs/1(C_SB) -> C_SB/1

== system Aircraft6dof_V2/Actuators - Plant /Equations Of Motion State Equations ==
  Fext_B : Inport
  Mext_B : Inport  Port=2
  omDot_motor : Inport  Port=3
  Earth Model : Subsystem
  MATLAB Function : MATLAB Function  Commented=on  TreatAsAtomicUnit=on
  Math Function : Math  Operator=transpose  SignedPower=on
  Product1 : Product  Multiplication=Matrix(*)
  Product2 : Product  Multiplication=Matrix(*)
  QUAT2ATT : Subsystem
  QUAT2DCM : Subsystem
  Rot Dyn (Moments) : Subsystem
  Rot Kin (Orientation) Euler : Subsystem  Commented=on
  Rot Kin (Orientation) Quaternion : Subsystem
  Trans Dyn (Forces) : Subsystem
  Trans Kin (Spherical) : Subsystem
  C_NB : Outport  VectorParamsAs1DForOutWhenUnconnected=off
  V_E_N_BE : Outport  Port=2  VectorParamsAs1DForOutWhenUnconnected=off
  ATT : Outport  Port=3  VectorParamsAs1DForOutWhenUnconnected=off
  accelMeasTrue : Outport  Port=4  VectorParamsAs1DForOutWhenUnconnected=off
  om_B_B_BE : Outport  Port=5  VectorParamsAs1DForOutWhenUnconnected=off
  C_BN : Outport  Port=6  VectorParamsAs1DForOutWhenUnconnected=off
  v_E_B_BE : Outport  Port=7  VectorParamsAs1DForOutWhenUnconnected=off
  p_E_E_BE : Outport  Port=8  VectorParamsAs1DForOutWhenUnconnected=off
  om_motor : Outport  Port=9  VectorParamsAs1DForOutWhenUnconnected=off
  wires:
  omDot_motor/1 -> Rot Dyn (Moments)/2(omDot_motor)
  Rot Dyn (Moments)/1(om_B_B_BE) -> Trans Dyn (Forces)/3(om_B_B_BE), Rot Kin (Orientation) Quaternion/1(om_B_B_BN), Rot Kin (Orientation) Euler/1(om_B_B_BN), om_B_B_BE/1
  Trans Dyn (Forces)/1(xDot_E_B_BE) -> Trans Kin (Spherical)/1(v_E_B_BE), v_E_B_BE/1, Product1/2
  Rot Kin (Orientation) Quaternion/1(q_BN) -> QUAT2DCM/1(Quat), QUAT2ATT/1(q)
  QUAT2DCM/1(DCM) -> C_BN/1, Math Function/1, Product2/1  "C_BN"
  Mext_B/1 -> Rot Dyn (Moments)/1(Mext_B)
  Fext_B/1 -> Trans Dyn (Forces)/1(Fext_B)
  QUAT2ATT/1(ATT) -> MATLAB Function/1(ATT), ATT/1
  Trans Kin (Spherical)/1(p_E_E_BE) -> Earth Model/1(p_E_E_BE), p_E_E_BE/1
  Math Function/1 -> C_NB/1, Trans Kin (Spherical)/2(C_NB), Product1/1  "C_NB"
  Product1/1 -> V_E_N_BE/1
  Earth Model/2(g_N) -> Product2/2
  Product2/1 -> Trans Dyn (Forces)/2(g_B)
  Rot Dyn (Moments)/2(om_motor) -> om_motor/1
  Trans Dyn (Forces)/2(accelMeasCG) -> accelMeasTrue/1
  Earth Model/1(Rearth) -> Trans Kin (Spherical)/3(Rearth)

== system Aircraft6dof_V2/Actuators - Plant /PropulsionForcesAndMoments ==
  dT_1_pct : Inport
  Om_Motor : Inport  Port=2
  v_B_BA : Inport  Port=3
  rho : Inport  Port=4
  Add : Sum  Inputs=++++
  Add1 : Sum  Inputs=++++
  Constant : Constant  Value=0
  Display1 : Display
  Display3 : Display
  PropulsionSystem1 : Subsystem
  Fprop_B : Outport  VectorParamsAs1DForOutWhenUnconnected=off
  Mprop_B : Outport  Port=2  VectorParamsAs1DForOutWhenUnconnected=off
  omDot : Outport  Port=3  VectorParamsAs1DForOutWhenUnconnected=off
  wires:
  dT_1_pct/1 -> PropulsionSystem1/4(u_p#_pct)
  Add/1 -> Fprop_B/1, Display3/1
  Add1/1 -> Mprop_B/1, Display1/1
  Constant/1 -> Add1/4, Add1/3, Add1/2, Add/4, Add/3, Add/2
  PropulsionSystem1/1(Fs4_B) -> Add/1
  rho/1 -> PropulsionSystem1/3(rho)
  v_B_BA/1 -> PropulsionSystem1/2(v_B_BA)
  Om_Motor/1 -> PropulsionSystem1/1(Om_p1)
  PropulsionSystem1/2(Ms4_B) -> Add1/1
  PropulsionSystem1/3(omDot) -> omDot/1

== system Aircraft6dof_V2/Actuators - Plant /Real Time Option ==
  Timer for Real-Time : S-Function  FunctionName=sfun_RealTimeOptional  Parameters=RatioToRealTime  SFunctionDeploymentMode=off  EnableBusSupport=off
  Excess Time but still not right : Outport  VectorParamsAs1DForOutWhenUnconnected=off
  wires:
  Timer for Real-Time/1 -> Excess Time but still not right/1

== system Aircraft6dof_V2/Controller/ControlMixer_A8 ==
  dA : Inport
  dF : Inport  Port=2
  dE : Inport  Port=3
  dR : Inport  Port=4
  dT : Inport  Port=5
  Constant1 : Constant  Value=A8.trim.MixMatrix
  Demux : Demux
  Mux1 : Mux
  Product1 : Product  Multiplication=Matrix(*)
  Sum{,1,3..4} (4 alike) : Sum  Inputs=|++
  trim_dE : Constant  Value=A8.trim.dE0
  trim_dEL : Constant  Value=A8.trim.dEL0
  trim_dER : Constant  Value=A8.trim.dER0
  trim_dR : Constant  Value=A8.trim.dR0
  dERcmd : Outport  VectorParamsAs1DForOutWhenUnconnected=off
  dELcmd : Outport  Port=2  VectorParamsAs1DForOutWhenUnconnected=off
  dElevcmd : Outport  Port=3  VectorParamsAs1DForOutWhenUnconnected=off
  dRudcmd : Outport  Port=4  VectorParamsAs1DForOutWhenUnconnected=off
  dTcmd : Outport  Port=5
  wires:
  trim_dE/1 -> Sum3/2
  dA/1 -> Mux1/1
  Constant1/1 -> Product1/1
  dF/1 -> Mux1/2
  dE/1 -> Mux1/3
  Mux1/1 -> Product1/2
  dR/1 -> Mux1/4
  dT/1 -> dTcmd/1
  trim_dEL/1 -> Sum1/2
  Product1/1 -> Demux/1
  trim_dER/1 -> Sum/2
  Demux/1 -> Sum/1
  Demux/2 -> Sum1/1
  Demux/3 -> Sum3/1
  Demux/4 -> Sum4/1
  trim_dR/1 -> Sum4/2
  Sum/1 -> dERcmd/1
  Sum1/1 -> dELcmd/1
  Sum3/1 -> dElevcmd/1
  Sum4/1 -> dRudcmd/1

== system Aircraft6dof_V2/Controller/LQR Controller ==
  attMeas : Inport
  ratesMeas : Inport  Port=2
  airDataMeas : Inport  Port=3
  attDes : Inport  Port=4
  ratesDes : Inport  Port=5
  airDataDes : Inport  Port=6
  1 if doing test : Constant  Value=A8.step.useCMDs
  Constant2 : Constant  Value=0
  Demux : Demux
  Demux{1..2,4..5} (4 alike) : Demux  Outputs=3
  LQR_Gain : Gain  Gain=-K_lqr_cmd  Multiplication=Matrix(K*u)
  Multiport Switch : MultiPortSwitch  Inputs=2  SaturateOnIntegerOverflow=off  InputSameDT=off
  Mux : Mux  Inputs=9
  Mux1 : Mux  Inputs=9
  Sum : Sum  Inputs=|+-
  Sum1 : Sum  Inputs=|++
  airdata_to_body_vel : MATLAB Function  TreatAsAtomicUnit=on
  airdata_to_body_vel1 : MATLAB Function  TreatAsAtomicUnit=on
  u_trim : Constant  Value=U_trim
  x_trim : Constant  Value=[Att_Trim; Vel_B_BA_Trim; Rates_Trim]
  dAil : Outport  VectorParamsAs1DForOutWhenUnconnected=off
  dFlap : Outport  Port=2  VectorParamsAs1DForOutWhenUnconnected=off
  dElev : Outport  Port=3  VectorParamsAs1DForOutWhenUnconnected=off
  dRud : Outport  Port=4  VectorParamsAs1DForOutWhenUnconnected=off
  dT : Outport  Port=5
  wires:
  Demux/4 -> dRud/1
  attMeas/1 -> Demux5/1
  Constant2/1 -> dT/1
  airDataMeas/1 -> airdata_to_body_vel/1(airdata)
  ratesMeas/1 -> Demux4/1
  Demux5/2 -> Mux/2  "theta"
  Demux5/1 -> Mux/1  "phi"
  Demux5/3 -> Mux/3  "psi"
  u_trim/1 -> Sum1/2
  Demux4/1 -> Mux/7  "P"
  Demux4/3 -> Mux/9  "R"
  Demux4/2 -> Mux/8  "Q"
  Mux/1 -> Sum/1
  Sum/1 -> LQR_Gain/1
  LQR_Gain/1 -> Sum1/1
  Sum1/1 -> Demux/1
  Demux/1 -> dAil/1
  Demux/2 -> dFlap/1
  Demux/3 -> dElev/1
  airdata_to_body_vel/1(u) -> Mux/4
  airdata_to_body_vel/2(v) -> Mux/5
  airdata_to_body_vel/3(w) -> Mux/6
  airdata_to_body_vel1/3(w) -> Mux1/6
  airdata_to_body_vel1/2(v) -> Mux1/5
  ratesDes/1 -> Demux1/1
  attDes/1 -> Demux2/1
  Demux1/3 -> Mux1/9  "R"
  Demux1/2 -> Mux1/8  "Q"
  Demux2/3 -> Mux1/3  "psi"
  Demux2/1 -> Mux1/1  "phi"
  Demux2/2 -> Mux1/2  "theta"
  airdata_to_body_vel1/1(u) -> Mux1/4
  Demux1/1 -> Mux1/7  "P"
  airDataDes/1 -> airdata_to_body_vel1/1(airdata)
  Multiport Switch/1 -> Sum/2
  1 if doing test/1 -> Multiport Switch/1
  x_trim/1 -> Multiport Switch/2
  Mux1/1 -> Multiport Switch/3

== system Aircraft6dof_V2/Controller/No Feedback Open Loop Commands Steps, Ramps, Sweeps, etc ==
  attDes : Inport
  ratesDes : Inport  Port=2
  airDataDes : Inport  Port=3
  accelDes : Inport  Port=4
  attMeas : Inport  Port=5
  ratesMeas : Inport  Port=6
  airDataMeas : Inport  Port=7
  accelMeas : Inport  Port=8
  Terminator{,1..7} (8 alike) : Terminator
  dAil_cmd_rad : Constant  Value=0
  dElev_cmd_rad : Constant  Value=0
  dFlap_cmd_rad : Constant  Value=0
  dRud_cmd_rad : Constant  Value=0
  dT_cmd : Constant  Value=0
  dAil : Outport  VectorParamsAs1DForOutWhenUnconnected=off
  dFlap : Outport  Port=2  VectorParamsAs1DForOutWhenUnconnected=off
  dElev : Outport  Port=3  VectorParamsAs1DForOutWhenUnconnected=off
  dRud : Outport  Port=4  VectorParamsAs1DForOutWhenUnconnected=off
  dT : Outport  Port=5
  wires:
  dAil_cmd_rad/1 -> dAil/1
  dElev_cmd_rad/1 -> dElev/1
  dFlap_cmd_rad/1 -> dFlap/1
  dRud_cmd_rad/1 -> dRud/1
  dT_cmd/1 -> dT/1
  accelMeas/1 -> Terminator7/1
  airDataMeas/1 -> Terminator6/1
  ratesMeas/1 -> Terminator5/1
  attMeas/1 -> Terminator4/1
  accelDes/1 -> Terminator3/1
  airDataDes/1 -> Terminator2/1
  ratesDes/1 -> Terminator1/1
  attDes/1 -> Terminator/1

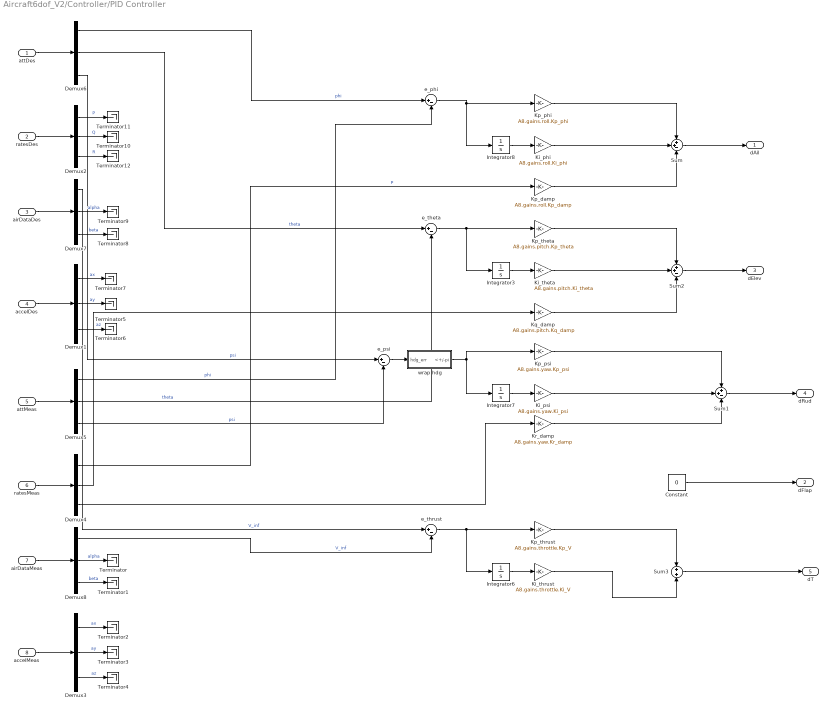
== system Aircraft6dof_V2/Controller/PID Controller ==
  attDes : Inport
  ratesDes : Inport  Port=2
  airDataDes : Inport  Port=3
  accelDes : Inport  Port=4
  attMeas : Inport  Port=5
  ratesMeas : Inport  Port=6
  airDataMeas : Inport  Port=7
  accelMeas : Inport  Port=8
  Constant : Constant  Value=0
  Demux{1..8} (8 alike) : Demux  Outputs=3
  Integrator{3,6..8} (4 alike) : Integrator
  Ki_phi : Gain  Gain=A8.gains.roll.Ki_phi
  Ki_psi : Gain  Gain=A8.gains.yaw.Ki_psi
  Ki_theta : Gain  Gain=A8.gains.pitch.Ki_theta
  Ki_thrust : Gain  Gain=A8.gains.throttle.Ki_V
  Kp_damp : Gain  Gain=A8.gains.roll.Kp_damp
  Kp_phi : Gain  Gain=A8.gains.roll.Kp_phi
  Kp_psi : Gain  Gain=A8.gains.yaw.Kp_psi
  Kp_theta : Gain  Gain=A8.gains.pitch.Kp_theta
  Kp_thrust : Gain  Gain=A8.gains.throttle.Kp_V
  Kq_damp : Gain  Gain=A8.gains.pitch.Kq_damp
  Kr_damp : Gain  Gain=A8.gains.yaw.Kr_damp
  Sum : Sum  Inputs=++-
  Sum1 : Sum  Inputs=++-
  Sum2 : Sum  Inputs=++-
  Sum3 : Sum
  Terminator{,1..12} (13 alike) : Terminator
  e_phi : Sum  Inputs=|+-
  e_psi : Sum  Inputs=|+-
  e_theta : Sum  Inputs=|+-
  e_thrust : Sum  Inputs=|+-
  wrap hdg : Subsystem
  dAil : Outport  VectorParamsAs1DForOutWhenUnconnected=off
  dFlap : Outport  Port=2  VectorParamsAs1DForOutWhenUnconnected=off
  dElev : Outport  Port=3  VectorParamsAs1DForOutWhenUnconnected=off
  dRud : Outport  Port=4  VectorParamsAs1DForOutWhenUnconnected=off
  dT : Outport  Port=5  VectorParamsAs1DForOutWhenUnconnected=off
  wires:
  Demux6/1 -> e_phi/1  "phi"
  Demux6/2 -> e_theta/1  "theta"
  Demux1/3 -> Terminator6/1  "az"
  Demux2/1 -> Terminator11/1  "P"
  Demux6/3 -> e_psi/1  "psi"
  airDataDes/1 -> Demux7/1
  Demux1/1 -> Terminator7/1  "ax"
  Demux1/2 -> Terminator5/1  "ay"
  accelDes/1 -> Demux1/1
  Demux2/3 -> Terminator12/1  "R"
  Demux7/3 -> Terminator8/1  "beta"
  ratesDes/1 -> Demux2/1
  Demux2/2 -> Terminator10/1  "Q"
  Demux7/2 -> Terminator9/1  "alpha"
  attDes/1 -> Demux6/1
  Demux7/1 -> e_thrust/1  "V_inf"
  attMeas/1 -> Demux5/1
  accelMeas/1 -> Demux3/1
  Demux3/2 -> Terminator3/1  "ay"
  Demux8/2 -> Terminator/1  "alpha"
  Demux8/3 -> Terminator1/1  "beta"
  Demux8/1 -> e_thrust/2  "V_inf"
  Demux3/3 -> Terminator4/1  "az"
  Demux5/2 -> e_theta/2  "theta"
  Demux3/1 -> Terminator2/1  "ax"
  Demux5/3 -> e_psi/2  "psi"
  ratesMeas/1 -> Demux4/1
  Demux5/1 -> e_phi/2  "phi"
  airDataMeas/1 -> Demux8/1
  Kp_phi/1 -> Sum/1
  Kp_psi/1 -> Sum1/1
  e_psi/1 -> wrap hdg/1(hdg_err)
  e_phi/1 -> Integrator8/1, Kp_phi/1
  e_thrust/1 -> Integrator6/1, Kp_thrust/1
  Sum3/1 -> dT/1
  Kp_thrust/1 -> Sum3/1
  Kp_damp/1 -> Sum/3
  e_theta/1 -> Integrator3/1, Kp_theta/1
  Kr_damp/1 -> Sum1/3
  Kp_theta/1 -> Sum2/1
  Kq_damp/1 -> Sum2/3
  Sum2/1 -> dElev/1
  Sum/1 -> dAil/1
  Sum1/1 -> dRud/1
  Constant/1 -> dFlap/1
  Ki_phi/1 -> Sum/2
  Ki_theta/1 -> Sum2/2
  Ki_psi/1 -> Sum1/2
  Ki_thrust/1 -> Sum3/2
  Integrator8/1 -> Ki_phi/1
  Integrator3/1 -> Ki_theta/1
  Integrator7/1 -> Ki_psi/1
  Integrator6/1 -> Ki_thrust/1
  Demux4/3 -> Kr_damp/1
  Demux4/2 -> Kq_damp/1
  Demux4/1 -> Kp_damp/1  "P"
  wrap hdg/1(<+/-pi) -> Integrator7/1, Kp_psi/1

== system Aircraft6dof_V2/Sensors/AccelSensor ==
  accelTrue : Inport
  Mux : Mux  Inputs=3
  Product : Product
  Sum : Sum  Inputs=+++
  ax : RandomNumber  Seed=A8.sensor.seed.accel  SampleTime=A8.sensor.sampleTime
  ay : RandomNumber  Seed=A8.sensor.seed.accel + 1  SampleTime=A8.sensor.sampleTime
  az : RandomNumber  Seed=A8.sensor.seed.accel + 2  SampleTime=A8.sensor.sampleTime
  bias : Constant  Value=A8.sensor.accel.bias
  sigma : Constant  Value=A8.sensor.accel.sigma
  accelMeas : Outport
  wires:
  ax/1 -> Mux/1
  accelTrue/1 -> Sum/3
  ay/1 -> Mux/2
  az/1 -> Mux/3
  sigma/1 -> Product/1
  bias/1 -> Sum/2
  Mux/1 -> Product/2
  Product/1 -> Sum/1
  Sum/1 -> accelMeas/1

== system Aircraft6dof_V2/Sensors/AirDataSensor ==
  w_B_BA : Inport
  Mux : Mux  Inputs=3
  Product : Product
  Sum : Sum  Inputs=+++
  Vinf_rnd : RandomNumber  Seed=A8.sensor.seed.airdata  SampleTime=A8.sensor.sampleTime
  alpha_rnd : RandomNumber  Seed=A8.sensor.seed.airdata + 1  SampleTime=A8.sensor.sampleTime
  beta_rnd : RandomNumber  Seed=A8.sensor.seed.airdata + 2  SampleTime=A8.sensor.sampleTime
  bias : Constant  Value=A8.sensor.airdata.bias
  sigma : Constant  Value=A8.sensor.airdata.sigma
  airdataMeas : Outport
  wires:
  Vinf_rnd/1 -> Mux/1
  w_B_BA/1 -> Sum/3
  Product/1 -> Sum/1
  alpha_rnd/1 -> Mux/2
  beta_rnd/1 -> Mux/3
  sigma/1 -> Product/1
  Mux/1 -> Product/2
  bias/1 -> Sum/2
  Sum/1 -> airdataMeas/1

== system Aircraft6dof_V2/Sensors/AttitudeSensor ==
  attTrue : Inport
  Mux : Mux  Inputs=3
  Product : Product
  Sum : Sum  Inputs=+++
  bias : Constant  Value=A8.sensor.att.bias
  phi : RandomNumber  Seed=A8.sensor.seed.att  SampleTime=A8.sensor.sampleTime
  psi : RandomNumber  Seed=A8.sensor.seed.att + 2  SampleTime=A8.sensor.sampleTime
  sigma : Constant  Value=A8.sensor.att.sigma
  theta : RandomNumber  Seed=A8.sensor.seed.att + 1  SampleTime=A8.sensor.sampleTime
  attMeas : Outport
  wires:
  attTrue/1 -> Sum/3
  phi/1 -> Mux/1
  theta/1 -> Mux/2
  Product/1 -> Sum/1
  psi/1 -> Mux/3
  Mux/1 -> Product/2
  sigma/1 -> Product/1
  bias/1 -> Sum/2
  Sum/1 -> attMeas/1

== system Aircraft6dof_V2/Sensors/GPSSensor ==
  posTrue : Inport
  velTrue : Inport  Port=2
  Mux : Mux  Inputs=3
  Product : Product
  Sum : Sum  Inputs=+++
  alt : RandomNumber  Seed=A8.sensor.seed.gpsPos + 2  SampleTime=A8.sensor.sampleTime
  bias : Constant  Value=A8.sensor.gps.posBias
  lat : RandomNumber  Seed=A8.sensor.seed.gpsPos  SampleTime=A8.sensor.sampleTime
  lon : RandomNumber  Seed=A8.sensor.seed.gpsPos + 1  SampleTime=A8.sensor.sampleTime
  sigma : Constant  Value=A8.sensor.gps.posSigma
  gpsPosMeas : Outport
  gpsVelMeas : Outport  Port=2
  wires:
  lat/1 -> Mux/1
  bias/1 -> Sum/2
  velTrue/1 -> gpsVelMeas/1
  lon/1 -> Mux/2
  sigma/1 -> Product/1
  Sum/1 -> gpsPosMeas/1
  alt/1 -> Mux/3
  Mux/1 -> Product/2
  Product/1 -> Sum/1
  posTrue/1 -> Sum/3

== system Aircraft6dof_V2/Sensors/GyroSensor ==
  ratesTrue : Inport
  Mux : Mux  Inputs=3
  P : RandomNumber  Seed=A8.sensor.seed.gyro  SampleTime=A8.sensor.sampleTime
  Product : Product
  Q : RandomNumber  Seed=A8.sensor.seed.gyro + 1  SampleTime=A8.sensor.sampleTime
  R : RandomNumber  Seed=A8.sensor.seed.gyro + 2  SampleTime=A8.sensor.sampleTime
  Sum : Sum  Inputs=+++
  bias : Constant  Value=A8.sensor.gyro.bias
  sigma : Constant  Value=A8.sensor.gyro.sigma
  ratesMeas : Outport
  wires:
  P/1 -> Mux/1
  Q/1 -> Mux/2
  Product/1 -> Sum/1
  R/1 -> Mux/3
  sigma/1 -> Product/1
  Mux/1 -> Product/2
  Sum/1 -> ratesMeas/1
  bias/1 -> Sum/2
  ratesTrue/1 -> Sum/3

== system Aircraft6dof_V2/Sensors/MagSensor ==
  attTrue : Inport
  MATLAB Function : MATLAB Function  TreatAsAtomicUnit=on
  MATLAB Function1 : MATLAB Function  TreatAsAtomicUnit=on
  Mux : Mux  Inputs=3
  Product : Product
  Sum : Sum  Inputs=+++
  bias : Constant  Value=A8.sensor.mag.bias
  magField_NED : Constant  Value=A8.sensor.magField_NED
  mag_1 : RandomNumber  Seed=A8.sensor.seed.mag  SampleTime=A8.sensor.sampleTime
  mag_2 : RandomNumber  Seed=A8.sensor.seed.mag + 1  SampleTime=A8.sensor.sampleTime
  mag_3 : RandomNumber  Seed=A8.sensor.seed.mag + 2  SampleTime=A8.sensor.sampleTime
  sigma : Constant  Value=A8.sensor.mag.sigma
  magMeasBody : Outport
  magHdgMeas : Outport  Port=2
  wires:
  mag_1/1 -> Mux/1
  Mux/1 -> Product/2
  mag_2/1 -> Mux/2
  mag_3/1 -> Mux/3
  Product/1 -> Sum/1
  sigma/1 -> Product/1
  magField_NED/1 -> MATLAB Function/2(mag_N)
  attTrue/1 -> MATLAB Function1/2(att_rad), MATLAB Function/1(att_rad)
  bias/1 -> Sum/2
  MATLAB Function/1(mag_B) -> Sum/3, MATLAB Function1/1(mag_B)
  Sum/1 -> magMeasBody/1
  MATLAB Function1/1(psi_mag) -> magHdgMeas/1

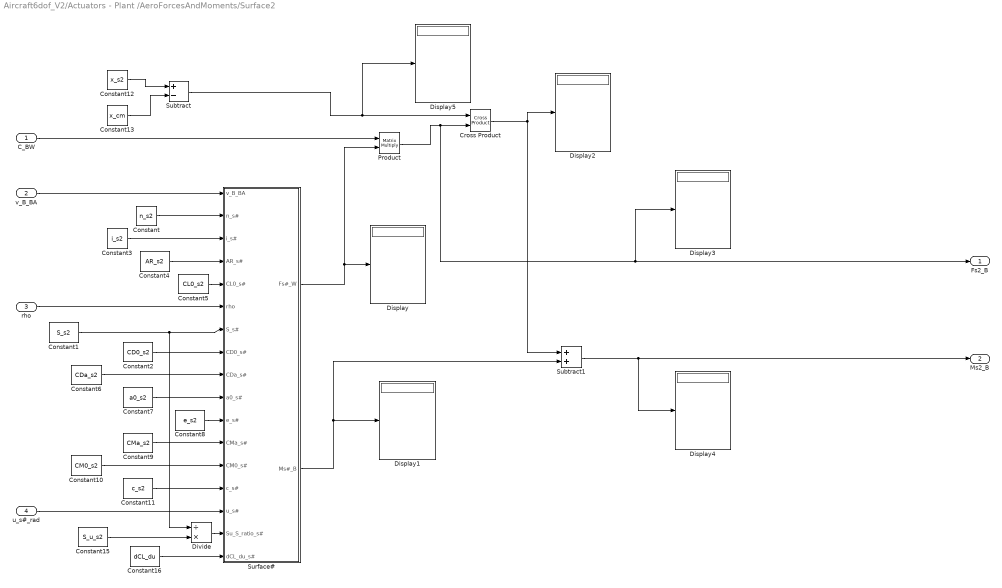
== system Aircraft6dof_V2/Actuators - Plant /AeroForcesAndMoments/Surface2 ==
  C_BW : Inport
  v_B_BA : Inport  Port=2
  rho : Inport  Port=3
  u_s#_rad : Inport  Port=4
  Constant : Constant  Value=n_s2
  Constant1 : Constant  Value=S_s2
  Constant10 : Constant  Value=CM0_s2
  Constant11 : Constant  Value=c_s2
  Constant12 : Constant  Value=x_s2
  Constant13 : Constant  Value=x_cm
  Constant15 : Constant  Value=S_u_s2
  Constant16 : Constant  Value=dCL_du
  Constant2 : Constant  Value=CD0_s2
  Constant3 : Constant  Value=i_s2
  Constant4 : Constant  Value=AR_s2
  Constant5 : Constant  Value=CL0_s2
  Constant6 : Constant  Value=CDa_s2
  Constant7 : Constant  Value=a0_s2
  Constant8 : Constant  Value=e_s2
  Constant9 : Constant  Value=CMa_s2
  Cross Product : vrlib/Utilities/Cross Product
  Display{,1..5} (6 alike) : Display
  Divide : Product  Inputs=/*
  Product : Product  Multiplication=Matrix(*)
  Subtract : Sum  Inputs=+-
  Subtract1 : Sum
  Surface# : Subsystem
  Fs2_B : Outport  VectorParamsAs1DForOutWhenUnconnected=off
  Ms2_B : Outport  Port=2  VectorParamsAs1DForOutWhenUnconnected=off
  wires:
  Subtract/1 -> Display5/1, Cross Product/1
  C_BW/1 -> Product/1
  Constant12/1 -> Subtract/1
  Constant13/1 -> Subtract/2
  Cross Product/1 -> Subtract1/1, Display2/1
  Product/1 -> Fs2_B/1, Display3/1, Cross Product/2
  Subtract1/1 -> Ms2_B/1, Display4/1
  Surface#/2(Ms#_B) -> Subtract1/2, Display1/1
  Constant10/1 -> Surface#/13(CM0_s#)
  Surface#/1(Fs#_W) -> Product/2, Display/1
  Constant11/1 -> Surface#/14(c_s#)
  Constant9/1 -> Surface#/12(CMa_s#)
  Constant7/1 -> Surface#/10(a0_s#)
  v_B_BA/1 -> Surface#/1(v_B_BA)
  Constant/1 -> Surface#/2(n_s#)
  Constant3/1 -> Surface#/3(i_s#)
  Constant4/1 -> Surface#/4(AR_s#)
  Constant5/1 -> Surface#/5(CL0_s#)
  rho/1 -> Surface#/6(rho)
  Constant2/1 -> Surface#/8(CD0_s#)
  Constant6/1 -> Surface#/9(CDa_s#)
  Constant8/1 -> Surface#/11(e_s#)
  Constant1/1 -> Divide/1, Surface#/7(S_s#)
  u_s#_rad/1 -> Surface#/15(u_s#)
  Constant15/1 -> Divide/2
  Constant16/1 -> Surface#/17(dCL_du_s#)
  Divide/1 -> Surface#/16(Su_S_ratio_s#)

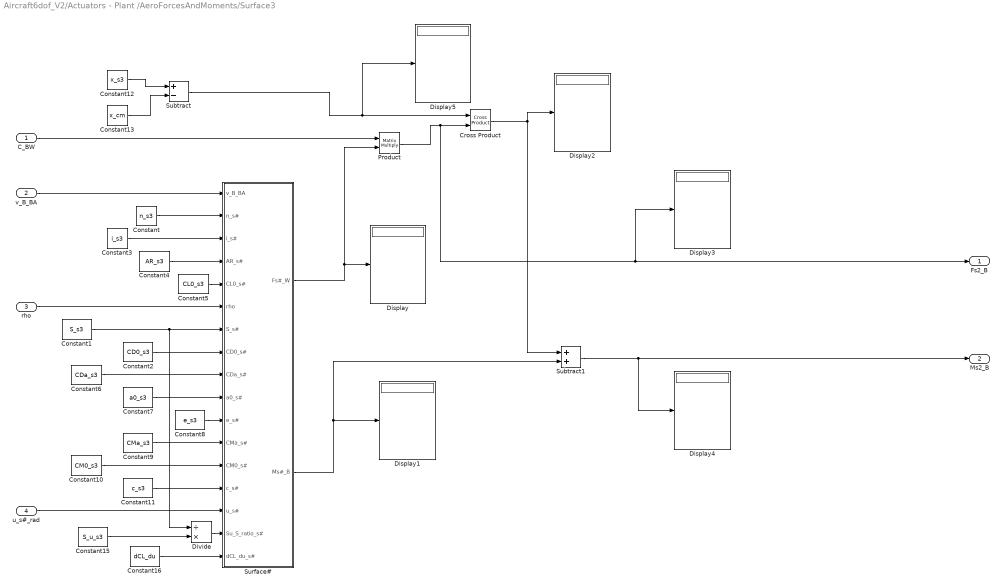
== system Aircraft6dof_V2/Actuators - Plant /AeroForcesAndMoments/Surface3 ==
  C_BW : Inport
  v_B_BA : Inport  Port=2
  rho : Inport  Port=3
  u_s#_rad : Inport  Port=4
  Constant : Constant  Value=n_s3
  Constant1 : Constant  Value=S_s3
  Constant10 : Constant  Value=CM0_s3
  Constant11 : Constant  Value=c_s3
  Constant12 : Constant  Value=x_s3
  Constant13 : Constant  Value=x_cm
  Constant15 : Constant  Value=S_u_s3
  Constant16 : Constant  Value=dCL_du
  Constant2 : Constant  Value=CD0_s3
  Constant3 : Constant  Value=i_s3
  Constant4 : Constant  Value=AR_s3
  Constant5 : Constant  Value=CL0_s3
  Constant6 : Constant  Value=CDa_s3
  Constant7 : Constant  Value=a0_s3
  Constant8 : Constant  Value=e_s3
  Constant9 : Constant  Value=CMa_s3
  Cross Product : vrlib/Utilities/Cross Product
  Display{,1..5} (6 alike) : Display
  Divide : Product  Inputs=/*
  Product : Product  Multiplication=Matrix(*)
  Subtract : Sum  Inputs=+-
  Subtract1 : Sum
  Surface# : Subsystem
  Fs2_B : Outport  VectorParamsAs1DForOutWhenUnconnected=off
  Ms2_B : Outport  Port=2  VectorParamsAs1DForOutWhenUnconnected=off
  wires:
  Subtract/1 -> Display5/1, Cross Product/1
  C_BW/1 -> Product/1
  Constant12/1 -> Subtract/1
  Constant13/1 -> Subtract/2
  Cross Product/1 -> Subtract1/1, Display2/1
  Product/1 -> Fs2_B/1, Display3/1, Cross Product/2
  Subtract1/1 -> Ms2_B/1, Display4/1
  Surface#/2(Ms#_B) -> Subtract1/2, Display1/1
  Constant10/1 -> Surface#/13(CM0_s#)
  Surface#/1(Fs#_W) -> Product/2, Display/1
  Constant11/1 -> Surface#/14(c_s#)
  Constant9/1 -> Surface#/12(CMa_s#)
  Constant7/1 -> Surface#/10(a0_s#)
  v_B_BA/1 -> Surface#/1(v_B_BA)
  Constant/1 -> Surface#/2(n_s#)
  Constant3/1 -> Surface#/3(i_s#)
  Constant4/1 -> Surface#/4(AR_s#)
  Constant5/1 -> Surface#/5(CL0_s#)
  rho/1 -> Surface#/6(rho)
  Constant2/1 -> Surface#/8(CD0_s#)
  Constant6/1 -> Surface#/9(CDa_s#)
  Constant8/1 -> Surface#/11(e_s#)
  Constant1/1 -> Divide/1, Surface#/7(S_s#)
  u_s#_rad/1 -> Surface#/15(u_s#)
  Constant15/1 -> Divide/2
  Constant16/1 -> Surface#/17(dCL_du_s#)
  Divide/1 -> Surface#/16(Su_S_ratio_s#)

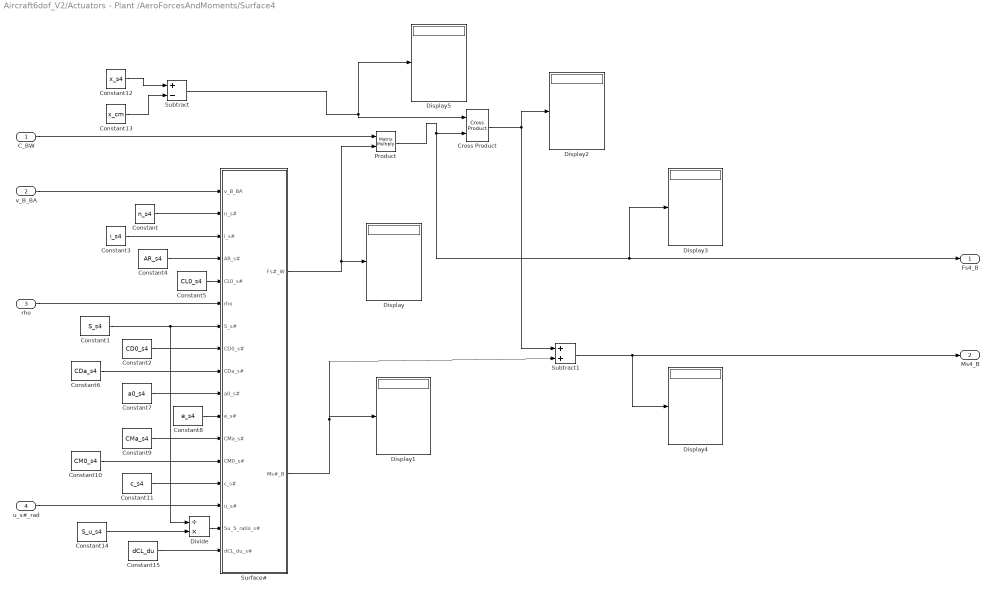
== system Aircraft6dof_V2/Actuators - Plant /AeroForcesAndMoments/Surface4 ==
  C_BW : Inport
  v_B_BA : Inport  Port=2
  rho : Inport  Port=3
  u_s#_rad : Inport  Port=4
  Constant : Constant  Value=n_s4
  Constant1 : Constant  Value=S_s4
  Constant10 : Constant  Value=CM0_s4
  Constant11 : Constant  Value=c_s4
  Constant12 : Constant  Value=x_s4
  Constant13 : Constant  Value=x_cm
  Constant14 : Constant  Value=S_u_s4
  Constant15 : Constant  Value=dCL_du
  Constant2 : Constant  Value=CD0_s4
  Constant3 : Constant  Value=i_s4
  Constant4 : Constant  Value=AR_s4
  Constant5 : Constant  Value=CL0_s4
  Constant6 : Constant  Value=CDa_s4
  Constant7 : Constant  Value=a0_s4
  Constant8 : Constant  Value=e_s4
  Constant9 : Constant  Value=CMa_s4
  Cross Product : vrlib/Utilities/Cross Product
  Display{,1..5} (6 alike) : Display
  Divide : Product  Inputs=/*
  Product : Product  Multiplication=Matrix(*)
  Subtract : Sum  Inputs=+-
  Subtract1 : Sum
  Surface# : Subsystem
  Fs4_B : Outport  VectorParamsAs1DForOutWhenUnconnected=off
  Ms4_B : Outport  Port=2  VectorParamsAs1DForOutWhenUnconnected=off
  wires:
  Subtract/1 -> Display5/1, Cross Product/1
  C_BW/1 -> Product/1
  Constant12/1 -> Subtract/1
  Constant13/1 -> Subtract/2
  Cross Product/1 -> Display2/1, Subtract1/1
  Product/1 -> Fs4_B/1, Display3/1, Cross Product/2
  Subtract1/1 -> Ms4_B/1, Display4/1
  Surface#/2(Ms#_B) -> Subtract1/2, Display1/1
  Constant10/1 -> Surface#/13(CM0_s#)
  Surface#/1(Fs#_W) -> Product/2, Display/1
  Constant11/1 -> Surface#/14(c_s#)
  Constant9/1 -> Surface#/12(CMa_s#)
  Constant7/1 -> Surface#/10(a0_s#)
  v_B_BA/1 -> Surface#/1(v_B_BA)
  Constant/1 -> Surface#/2(n_s#)
  Constant3/1 -> Surface#/3(i_s#)
  Constant4/1 -> Surface#/4(AR_s#)
  Constant5/1 -> Surface#/5(CL0_s#)
  rho/1 -> Surface#/6(rho)
  Constant1/1 -> Divide/1, Surface#/7(S_s#)
  Constant2/1 -> Surface#/8(CD0_s#)
  Constant6/1 -> Surface#/9(CDa_s#)
  Constant8/1 -> Surface#/11(e_s#)
  u_s#_rad/1 -> Surface#/15(u_s#)
  Divide/1 -> Surface#/16(Su_S_ratio_s#)
  Constant14/1 -> Divide/2
  Constant15/1 -> Surface#/17(dCL_du_s#)
